simulink model "MicrostrainIMUTest02"  (R2013a)
settings: Solver=FixedStepDiscrete  StartTime=0.0  StopTime=inf  FixedStep=0.001  RelTol=1e-3
undefined symbols (not defined in the file or in its folder): IMU_Alignment_Params, KVHOrientationCal, m_XR17D15x, MicrostrainOrientationCal, standard, XOFF, XON
libraries: speedgoatlib x26, xpcethercatlib x25, xpcseriallib x13, simulink x5, dspswit3 x1, xpclib x1
(part 1 of 2)
settings Model: xpc_rtwmakecfg_data=_xpcethercatlib_  BufferReuse=off  Creator=bgbuss  LastModifiedBy=bgbuss
settings DataIOCC: LimitDataPoints=off
settings OptimizationCC: BlockReduction=off  OptimizeBlockIOStorage=off  BufferReuse=off  ExpressionFolding=off  LocalBlockOutputs=off
settings DebuggingCC: UnderspecifiedInitializationDetection=Simplified
settings HardwareCC: ProdIntDivRoundTo=Zero  ProdEndianess=LittleEndian  ProdHWDeviceType=Generic->32-bit x86 compatible
settings RTWCC: SystemTargetFile=xpctarget.tlc  TemplateMakefile=xpc_default_tmf  Description=xPC Target  ProcessScript=xpctarget_make_rtw_hook  RTWCompilerOptimization=On
settings xpcTargetCC: TargetFcnLib=ansi_tfl_table_tmw.mat  CodeReplacementLibrary=XPC_BLAS  ParMdlRefBuildCompliant=on  ConcurrentExecutionCompliant=on  CombineSignalStateStructs=off  MATLABClassNameForMDSCustomization=xpcAperiodicCustomization  GRTInterface=on  GenerateAllocFcn=off  RL32LogBufSizeModifier=100000000  xPCTaskExecutionProfile=off  xPCRL32EventNumber=5000  xPCisModelTimeout=off  xPCModelTimeoutSecs=20  xPCLoadParamSetFile=off  xPCConcurrentTasks=off  xPCEnableSFAnimation=off

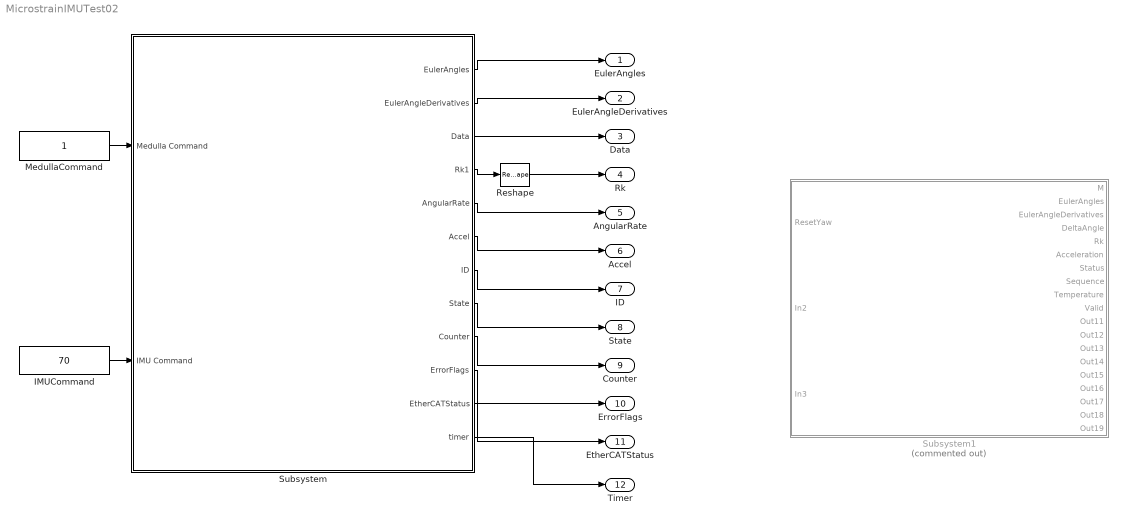
== system MicrostrainIMUTest02 ==
  IMUCommand : Constant  Value=70
  MedullaCommand : Constant
  Reshape : Reshape
  Subsystem : Subsystem
  Subsystem1 : Subsystem  Commented=on
  EulerAngles : Outport
  EulerAngleDerivatives : Outport  Port=2
  Data : Outport  Port=3
  Rk : Outport  Port=4
  AngularRate : Outport  Port=5
  Accel : Outport  Port=6
  ID : Outport  Port=7
  State : Outport  Port=8
  Counter : Outport  Port=9
  ErrorFlags : Outport  Port=10
  EtherCATStatus : Outport  Port=11
  Timer : Outport  Port=12
  wires:
  MedullaCommand/1 -> Subsystem/1(Medulla Command)
  IMUCommand/1 -> Subsystem/2(IMU Command)
  Subsystem/11(EtherCATStatus) -> EtherCATStatus/1
  Subsystem/1(EulerAngles) -> EulerAngles/1
  Subsystem/2(EulerAngleDerivatives) -> EulerAngleDerivatives/1
  Subsystem/3(Data) -> Data/1
  Subsystem/4(Rk1) -> Reshape/1
  Subsystem/5(AngularRate) -> AngularRate/1
  Subsystem/6(Accel) -> Accel/1
  Subsystem/7(ID) -> ID/1
  Subsystem/8(State) -> State/1
  Subsystem/9(Counter) -> Counter/1
  Subsystem/10(ErrorFlags) -> ErrorFlags/1
  Reshape/1 -> Rk/1
  Subsystem/12(timer) -> Timer/1

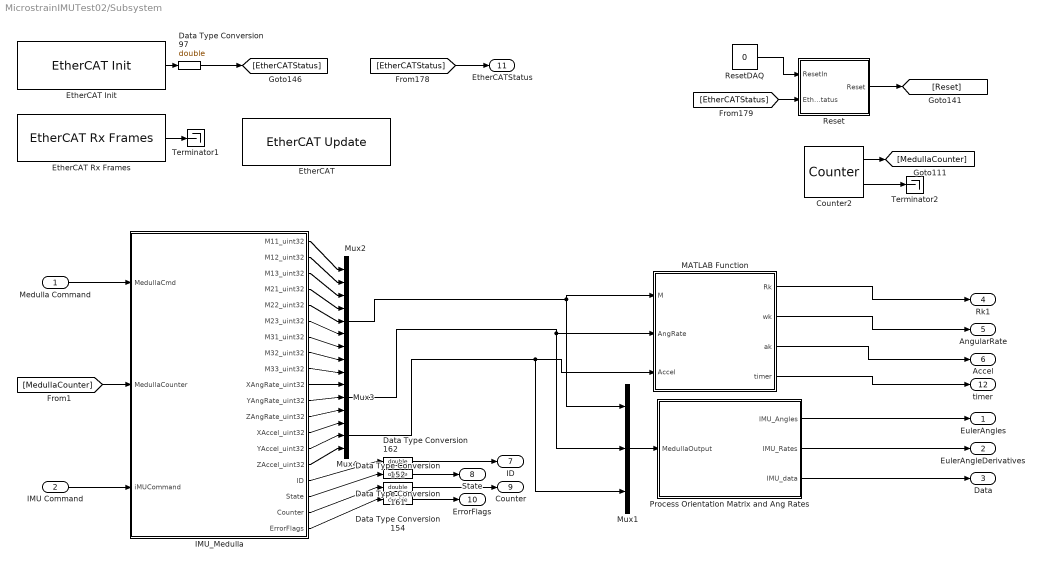
== system MicrostrainIMUTest02/Subsystem ==
  Medulla Command : Inport
  IMU Command : Inport  Port=2
  Counter2 : dspswit3/Counter  Direction=Up  CountEvent=Free running  CounterSize=User defined  MaxCount=65535  InitialCount=0  Output=Count and Hit  HitValue=32  ResetInput=off  SamplesPerFrame=1  Ts=.001  CntDtype=double  HitDtype=Logical
  Data Type Conversion{97,152,154,161..162} (5 alike) : DataTypeConversion  OutDataTypeStr=double
  EtherCAT : xpcethercatlib/EtherCAT Update   Priority=4  device_id=0  task_id_list=[1]  task_rates=[1]  task_priorities=[1500]
  EtherCAT Init : xpcethercatlib/EtherCAT Init   Priority=0  config_file='microstrain-imu-box07-eni.xml'  device_id=0  pci_bus=7  pci_slot=0  enaDC=on  errRptLevel=0  sample_time=0.001000
  EtherCAT Rx Frames : xpcethercatlib/EtherCAT Rx Frames   Priority=1  device_id=0  sample_time=0
  IMU_Medulla : Subsystem
  MATLAB Function : MATLAB Function  TreatAsAtomicUnit=on
  Mux1 : Mux  Inputs=3
  Mux2 : Mux  Inputs=9
  Mux3 : Mux  Inputs=3
  Mux4 : Mux  Inputs=3
  Process Orientation Matrix and Ang Rates : Subsystem
  Reset : Subsystem
  ResetDAQ : Constant  Value=0
  Terminator1 : Terminator
  Terminator2 : Terminator
  EulerAngles : Outport
  EulerAngleDerivatives : Outport  Port=2
  Data : Outport  Port=3
  Rk1 : Outport  Port=4
  AngularRate : Outport  Port=5
  Accel : Outport  Port=6
  ID : Outport  Port=7
  State : Outport  Port=8
  Counter : Outport  Port=9
  ErrorFlags : Outport  Port=10
  EtherCATStatus : Outport  Port=11
  timer : Outport  Port=12
  wires:
  IMU_Medulla/3(M13_uint32) -> Mux2/3
  IMU_Medulla/19(ErrorFlags) -> Data Type Conversion154/1
  IMU_Medulla/9(M33_uint32) -> Mux2/9
  IMU_Medulla/11(YAngRate_uint32) -> Mux3/2
  IMU_Medulla/15(ZAccel_uint32) -> Mux4/3
  [MedullaCounter] -> IMU_Medulla/2(MedullaCounter)
  IMU_Medulla/12(ZAngRate_uint32) -> Mux3/3
  IMU_Medulla/1(M11_uint32) -> Mux2/1
  IMU_Medulla/5(M22_uint32) -> Mux2/5
  IMU_Medulla/10(XAngRate_uint32) -> Mux3/1
  IMU_Medulla/14(YAccel_uint32) -> Mux4/2
  IMU_Medulla/13(XAccel_uint32) -> Mux4/1
  Data Type Conversion161/1 -> State/1
  IMU_Medulla/8(M32_uint32) -> Mux2/8
  Data Type Conversion162/1 -> ID/1
  IMU_Medulla/2(M12_uint32) -> Mux2/2
  IMU_Medulla/16(ID) -> Data Type Conversion162/1
  IMU_Medulla/6(M23_uint32) -> Mux2/6
  IMU_Medulla/4(M21_uint32) -> Mux2/4
  IMU_Medulla/7(M31_uint32) -> Mux2/7
  IMU_Medulla/18(Counter) -> Data Type Conversion152/1
  IMU_Medulla/17(State) -> Data Type Conversion161/1
  Mux3/1 -> Mux1/2, MATLAB Function/2(AngRate)
  Mux1/1 -> Process Orientation Matrix and Ang Rates/1(MedullaOutput)
  Process Orientation Matrix and Ang Rates/1(IMU_Angles) -> EulerAngles/1
  Process Orientation Matrix and Ang Rates/2(IMU_Rates) -> EulerAngleDerivatives/1
  Process Orientation Matrix and Ang Rates/3(IMU_data) -> Data/1
  [EtherCATStatus] -> EtherCATStatus/1
  ResetDAQ/1 -> Reset/1(ResetIn)
  Counter2/1 -> [MedullaCounter]
  [EtherCATStatus] -> Reset/2(EtherCATStatus)
  Reset/1(Reset) -> [Reset]
  Counter2/2 -> Terminator2/1
  Data Type Conversion97/1 -> [EtherCATStatus]
  EtherCAT Init/1 -> Data Type Conversion97/1
  EtherCAT Rx Frames/1 -> Terminator1/1
  Mux4/1 -> Mux1/3, MATLAB Function/3(Accel)
  Mux2/1 -> Mux1/1, MATLAB Function/1(M)
  Data Type Conversion152/1 -> Counter/1
  Data Type Conversion154/1 -> ErrorFlags/1
  Medulla Command/1 -> IMU_Medulla/1(MedullaCmd)
  IMU Command/1 -> IMU_Medulla/3(iMUCommand)
  MATLAB Function/1(Rk) -> Rk1/1
  MATLAB Function/2(wk) -> AngularRate/1
  MATLAB Function/3(ak) -> Accel/1
  MATLAB Function/4(timer) -> timer/1

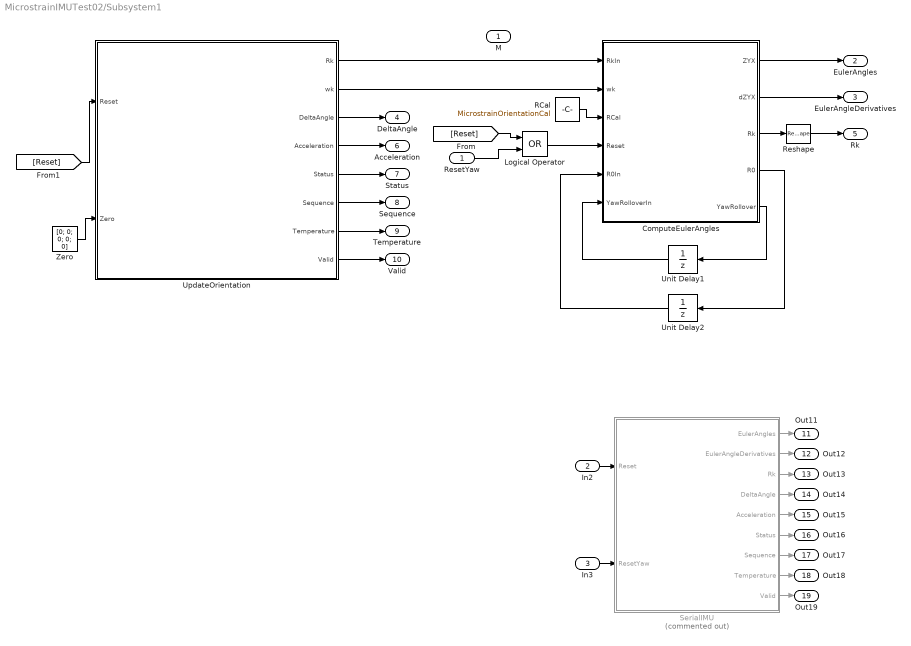
== system MicrostrainIMUTest02/Subsystem1 ==
  ResetYaw : Inport
  In2 : Inport  Port=2
  In3 : Inport  Port=3
  ComputeEulerAngles : MATLAB Function  TreatAsAtomicUnit=on
  Logical Operator : Logic  Operator=OR  AllPortsSameDT=off  OutDataTypeStr=boolean
  RCal : Constant  Value=MicrostrainOrientationCal
  Reshape : Reshape
  SerialIMU : Subsystem  Commented=on
  Unit Delay1 : UnitDelay  InitialCondition=[0; 0]  SampleTime=-1
  Unit Delay2 : UnitDelay  InitialCondition=zeros(3,3)  SampleTime=-1
  UpdateOrientation : Subsystem
  Zero : Constant  Value=[0; 0; 0; 0; 0]
  M : Outport
  EulerAngles : Outport  Port=2
  EulerAngleDerivatives : Outport  Port=3
  DeltaAngle : Outport  Port=4
  Rk : Outport  Port=5
  Acceleration : Outport  Port=6
  Status : Outport  Port=7
  Sequence : Outport  Port=8
  Temperature : Outport  Port=9
  Valid : Outport  Port=10
  Out11 : Outport  Port=11
  Out12 : Outport  Port=12
  Out13 : Outport  Port=13
  Out14 : Outport  Port=14
  Out15 : Outport  Port=15
  Out16 : Outport  Port=16
  Out17 : Outport  Port=17
  Out18 : Outport  Port=18
  Out19 : Outport  Port=19
  wires:
  SerialIMU/6(Status) -> Out16/1
  SerialIMU/8(Temperature) -> Out18/1
  In2/1 -> SerialIMU/1(Reset)
  SerialIMU/1(EulerAngles) -> Out11/1
  SerialIMU/3(Rk) -> Out13/1
  SerialIMU/5(Acceleration) -> Out15/1
  SerialIMU/2(EulerAngleDerivatives) -> Out12/1
  SerialIMU/7(Sequence) -> Out17/1
  In3/1 -> SerialIMU/2(ResetYaw)
  SerialIMU/9(Valid) -> Out19/1
  SerialIMU/4(DeltaAngle) -> Out14/1
  ComputeEulerAngles/1(ZYX) -> EulerAngles/1
  Logical Operator/1 -> ComputeEulerAngles/4(Reset)
  ResetYaw/1 -> Logical Operator/2
  Unit Delay1/1 -> ComputeEulerAngles/6(YawRolloverIn)
  ComputeEulerAngles/5(YawRollover) -> Unit Delay1/1
  UpdateOrientation/2(wk) -> ComputeEulerAngles/2(wk)
  UpdateOrientation/1(Rk) -> ComputeEulerAngles/1(RkIn)
  Reshape/1 -> Rk/1
  [Reset] -> Logical Operator/1
  ComputeEulerAngles/3(Rk) -> Reshape/1
  ComputeEulerAngles/4(R0) -> Unit Delay2/1
  Unit Delay2/1 -> ComputeEulerAngles/5(R0In)
  RCal/1 -> ComputeEulerAngles/3(RCal)
  [Reset] -> UpdateOrientation/1(Reset)
  Zero/1 -> UpdateOrientation/2(Zero)
  UpdateOrientation/3(DeltaAngle) -> DeltaAngle/1
  UpdateOrientation/6(Sequence) -> Sequence/1
  UpdateOrientation/5(Status) -> Status/1
  UpdateOrientation/4(Acceleration) -> Acceleration/1
  UpdateOrientation/7(Temperature) -> Temperature/1
  UpdateOrientation/8(Valid) -> Valid/1
  ComputeEulerAngles/2(dZYX) -> EulerAngleDerivatives/1

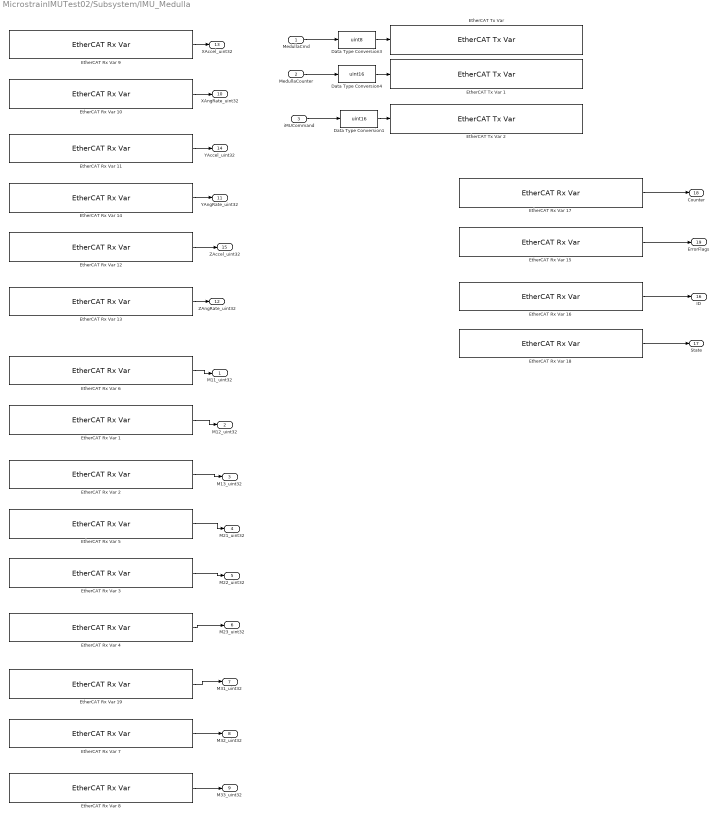
== system MicrostrainIMUTest02/Subsystem/IMU_Medulla ==
  MedullaCmd : Inport
  MedullaCounter : Inport  Port=2
  iMUCommand : Inport  Port=3
  Data Type Conversion1 : DataTypeConversion  OutDataTypeStr=uint16
  Data Type Conversion3 : DataTypeConversion  OutDataTypeStr=uint8
  Data Type Conversion4 : DataTypeConversion  OutDataTypeStr=uint16
  EtherCAT Rx Var 1 : xpcethercatlib/EtherCAT Rx Var   Priority=2  sig_name=Box 7 (ATRIAS 2.1 Microstrain IMU (Medulla 1.5)).M.M12  sig_offset=720  sig_type=uint32  type_size=32  sig_dim=1  device_id=0  sample_time=0.001000
  EtherCAT Rx Var 10 : xpcethercatlib/EtherCAT Rx Var   Priority=2  sig_name=Box 7 (ATRIAS 2.1 Microstrain IMU (Medulla 1.5)).Xaxes.XAngRate  sig_offset=496  sig_type=uint32  type_size=32  sig_dim=1  device_id=0  sample_time=0.001000
  EtherCAT Rx Var 11 : xpcethercatlib/EtherCAT Rx Var   Priority=2  sig_name=Box 7 (ATRIAS 2.1 Microstrain IMU (Medulla 1.5)).Yaxes.YAccel  sig_offset=592  sig_type=uint32  type_size=32  sig_dim=1  device_id=0  sample_time=0.001000
  EtherCAT Rx Var 12 : xpcethercatlib/EtherCAT Rx Var   Priority=2  sig_name=Box 7 (ATRIAS 2.1 Microstrain IMU (Medulla 1.5)).Zaxes.ZAccel  sig_offset=656  sig_type=uint32  type_size=32  sig_dim=1  device_id=0  sample_time=0.001000
  EtherCAT Rx Var 13 : xpcethercatlib/EtherCAT Rx Var   Priority=2  sig_name=Box 7 (ATRIAS 2.1 Microstrain IMU (Medulla 1.5)).Zaxes.ZAngRate  sig_offset=624  sig_type=uint32  type_size=32  sig_dim=1  device_id=0  sample_time=0.001000
  EtherCAT Rx Var 14 : xpcethercatlib/EtherCAT Rx Var   Priority=2  sig_name=Box 7 (ATRIAS 2.1 Microstrain IMU (Medulla 1.5)).Yaxes.YAngRate  sig_offset=560  sig_type=uint32  type_size=32  sig_dim=1  device_id=0  sample_time=0.001000
  EtherCAT Rx Var 15 : xpcethercatlib/EtherCAT Rx Var   Priority=2  sig_name=Box 7 (ATRIAS 2.1 Microstrain IMU (Medulla 1.5)).uController Status.Error Flags  sig_offset=488  sig_type=uint8  type_size=8  sig_dim=1  device_id=0  sample_time=0.001000
  EtherCAT Rx Var 16 : xpcethercatlib/EtherCAT Rx Var   Priority=2  sig_name=Box 7 (ATRIAS 2.1 Microstrain IMU (Medulla 1.5)).uController Status.ID  sig_offset=464  sig_type=uint8  type_size=8  sig_dim=1  device_id=0  sample_time=0.001000
  EtherCAT Rx Var 17 : xpcethercatlib/EtherCAT Rx Var   Priority=2  sig_name=Box 7 (ATRIAS 2.1 Microstrain IMU (Medulla 1.5)).uController Status.Counter  sig_offset=480  sig_type=uint8  type_size=8  sig_dim=1  device_id=0  sample_time=0.001000
  EtherCAT Rx Var 18 : xpcethercatlib/EtherCAT Rx Var   Priority=2  sig_name=Box 7 (ATRIAS 2.1 Microstrain IMU (Medulla 1.5)).uController Status.State  sig_offset=472  sig_type=uint8  type_size=8  sig_dim=1  device_id=0  sample_time=0.001000
  EtherCAT Rx Var 19 : xpcethercatlib/EtherCAT Rx Var   Priority=2  sig_name=Box 7 (ATRIAS 2.1 Microstrain IMU (Medulla 1.5)).M.M31  sig_offset=880  sig_type=uint32  type_size=32  sig_dim=1  device_id=0  sample_time=0.001000
  EtherCAT Rx Var 2 : xpcethercatlib/EtherCAT Rx Var   Priority=2  sig_name=Box 7 (ATRIAS 2.1 Microstrain IMU (Medulla 1.5)).M.M13  sig_offset=752  sig_type=uint32  type_size=32  sig_dim=1  device_id=0  sample_time=0.001000
  EtherCAT Rx Var 3 : xpcethercatlib/EtherCAT Rx Var   Priority=2  sig_name=Box 7 (ATRIAS 2.1 Microstrain IMU (Medulla 1.5)).M.M22  sig_offset=816  sig_type=uint32  type_size=32  sig_dim=1  device_id=0  sample_time=0.001000
  EtherCAT Rx Var 4 : xpcethercatlib/EtherCAT Rx Var   Priority=2  sig_name=Box 7 (ATRIAS 2.1 Microstrain IMU (Medulla 1.5)).M.M23  sig_offset=848  sig_type=uint32  type_size=32  sig_dim=1  device_id=0  sample_time=0.001000
  EtherCAT Rx Var 5 : xpcethercatlib/EtherCAT Rx Var   Priority=2  sig_name=Box 7 (ATRIAS 2.1 Microstrain IMU (Medulla 1.5)).M.M21  sig_offset=784  sig_type=uint32  type_size=32  sig_dim=1  device_id=0  sample_time=0.001000
  EtherCAT Rx Var 6 : xpcethercatlib/EtherCAT Rx Var   Priority=2  sig_name=Box 7 (ATRIAS 2.1 Microstrain IMU (Medulla 1.5)).M.M11  sig_offset=688  sig_type=uint32  type_size=32  sig_dim=1  device_id=0  sample_time=0.001000
  EtherCAT Rx Var 7 : xpcethercatlib/EtherCAT Rx Var   Priority=2  sig_name=Box 7 (ATRIAS 2.1 Microstrain IMU (Medulla 1.5)).M.M32  sig_offset=912  sig_type=uint32  type_size=32  sig_dim=1  device_id=0  sample_time=0.001000
  EtherCAT Rx Var 8 : xpcethercatlib/EtherCAT Rx Var   Priority=2  sig_name=Box 7 (ATRIAS 2.1 Microstrain IMU (Medulla 1.5)).M.M33  sig_offset=944  sig_type=uint32  type_size=32  sig_dim=1  device_id=0  sample_time=0.001000
  EtherCAT Rx Var 9 : xpcethercatlib/EtherCAT Rx Var   Priority=2  sig_name=Box 7 (ATRIAS 2.1 Microstrain IMU (Medulla 1.5)).Xaxes.XAccel  sig_offset=528  sig_type=uint32  type_size=32  sig_dim=1  device_id=0  sample_time=0.001000
  "EtherCAT Tx Var " : xpcethercatlib/EtherCAT Tx Var   Priority=3  sig_name=Box 7 (ATRIAS 2.1 Microstrain IMU (Medulla 1.5)).uControllerInput.Command  sig_offset=464  sig_type=uint8  type_size=8  sig_dim=1  device_id=0  sample_time=0.001000
  EtherCAT Tx Var 1 : xpcethercatlib/EtherCAT Tx Var   Priority=3  sig_name=Box 7 (ATRIAS 2.1 Microstrain IMU (Medulla 1.5)).uControllerInput.Counter  sig_offset=472  sig_type=uint16  type_size=16  sig_dim=1  device_id=0  sample_time=0.001000
  EtherCAT Tx Var 2 : xpcethercatlib/EtherCAT Tx Var   Priority=3  sig_name=Box 7 (ATRIAS 2.1 Microstrain IMU (Medulla 1.5)).uControllerInput.IMU_cmd  sig_offset=488  sig_type=uint16  type_size=16  sig_dim=1  device_id=0  sample_time=0.001000
  M11_uint32 : Outport
  M12_uint32 : Outport  Port=2
  M13_uint32 : Outport  Port=3
  M21_uint32 : Outport  Port=4
  M22_uint32 : Outport  Port=5
  M23_uint32 : Outport  Port=6
  M31_uint32 : Outport  Port=7
  M32_uint32 : Outport  Port=8
  M33_uint32 : Outport  Port=9
  XAngRate_uint32 : Outport  Port=10
  YAngRate_uint32 : Outport  Port=11
  ZAngRate_uint32 : Outport  Port=12
  XAccel_uint32 : Outport  Port=13
  YAccel_uint32 : Outport  Port=14
  ZAccel_uint32 : Outport  Port=15
  ID : Outport  Port=16
  State : Outport  Port=17
  Counter : Outport  Port=18
  ErrorFlags : Outport  Port=19
  wires:
  EtherCAT Rx Var 9/1 -> XAccel_uint32/1
  EtherCAT Rx Var 10/1 -> XAngRate_uint32/1
  EtherCAT Rx Var 11/1 -> YAccel_uint32/1
  EtherCAT Rx Var 14/1 -> YAngRate_uint32/1
  EtherCAT Rx Var 12/1 -> ZAccel_uint32/1
  EtherCAT Rx Var 13/1 -> ZAngRate_uint32/1
  EtherCAT Rx Var 6/1 -> M11_uint32/1
  EtherCAT Rx Var 1/1 -> M12_uint32/1
  EtherCAT Rx Var 2/1 -> M13_uint32/1
  EtherCAT Rx Var 5/1 -> M21_uint32/1
  EtherCAT Rx Var 3/1 -> M22_uint32/1
  EtherCAT Rx Var 4/1 -> M23_uint32/1
  EtherCAT Rx Var 19/1 -> M31_uint32/1
  EtherCAT Rx Var 7/1 -> M32_uint32/1
  EtherCAT Rx Var 8/1 -> M33_uint32/1
  Data Type Conversion3/1 -> "EtherCAT Tx Var "/1
  Data Type Conversion4/1 -> EtherCAT Tx Var 1/1
  MedullaCmd/1 -> Data Type Conversion3/1
  MedullaCounter/1 -> Data Type Conversion4/1
  iMUCommand/1 -> Data Type Conversion1/1
  Data Type Conversion1/1 -> EtherCAT Tx Var 2/1
  EtherCAT Rx Var 17/1 -> Counter/1
  EtherCAT Rx Var 15/1 -> ErrorFlags/1
  EtherCAT Rx Var 16/1 -> ID/1
  EtherCAT Rx Var 18/1 -> State/1

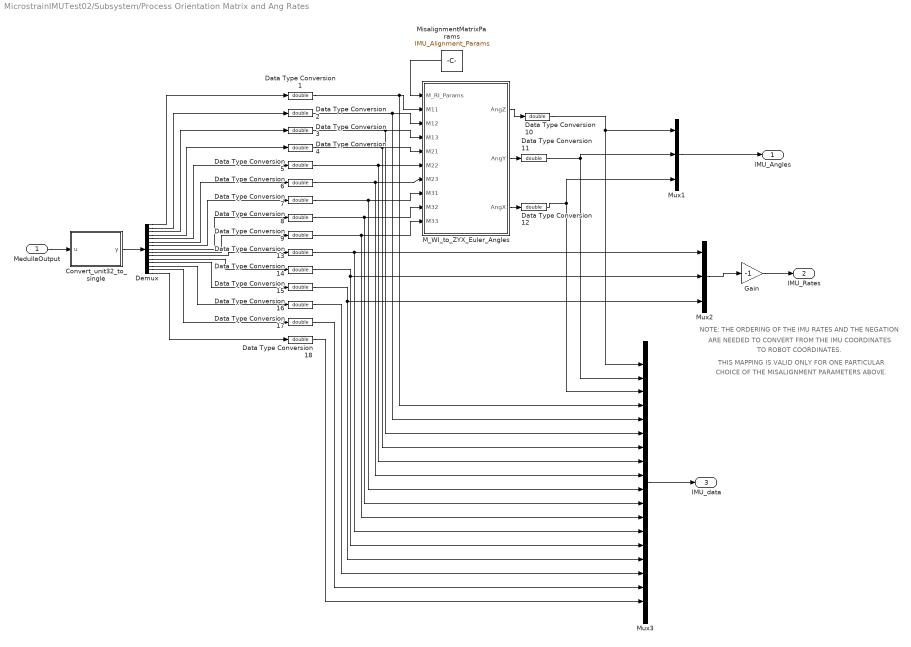
== system MicrostrainIMUTest02/Subsystem/Process Orientation Matrix and Ang Rates ==
  note: NOTE: THE ORDERING OF THE IMU RATES AND THE NEGATION
  note: ARE NEEDED TO CONVERT FROM THE IMU COORDINATES
  note: TO ROBOT COORDINATES.
  note: THIS MAPPING IS VALID ONLY FOR ONE PARTICULAR
  note: CHOICE OF THE MISALIGNMENT PARAMETERS ABOVE.
  MedullaOutput : Inport
  Convert_unit32_to_single : MATLAB Function  TreatAsAtomicUnit=on
  Data Type Conversion{1..18} (18 alike) : DataTypeConversion  OutDataTypeStr=double
  Demux : Demux  Outputs=15
  Gain : Gain  Gain=-1
  M_WI_to_ZYX_Euler_Angles : MATLAB Function  TreatAsAtomicUnit=on
  MisalignmentMatrixParams : Constant  Value=IMU_Alignment_Params
  Mux1 : Mux  Inputs=3
  Mux2 : Mux  Inputs=3
  Mux3 : Mux  Inputs=18
  IMU_Angles : Outport
  IMU_Rates : Outport  Port=2
  IMU_data : Outport  Port=3
  wires:
  Mux3/1 -> IMU_data/1
  Mux1/1 -> IMU_Angles/1
  Data Type Conversion16/1 -> Mux3/16
  Data Type Conversion17/1 -> Mux3/17
  Data Type Conversion18/1 -> Mux3/18
  Demux/15 -> Data Type Conversion18/1
  Demux/14 -> Data Type Conversion17/1
  Demux/13 -> Data Type Conversion16/1
  Demux/12 -> Data Type Conversion15/1
  Demux/11 -> Data Type Conversion14/1
  Demux/10 -> Data Type Conversion13/1
  Demux/9 -> Data Type Conversion9/1
  Demux/8 -> Data Type Conversion8/1
  Demux/7 -> Data Type Conversion7/1
  Demux/6 -> Data Type Conversion6/1
  Demux/5 -> Data Type Conversion5/1
  Demux/4 -> Data Type Conversion4/1
  Demux/3 -> Data Type Conversion3/1
  Demux/2 -> Data Type Conversion2/1
  Demux/1 -> Data Type Conversion1/1
  MisalignmentMatrixParams/1 -> M_WI_to_ZYX_Euler_Angles/1(M_RI_Params)
  Data Type Conversion15/1 -> Mux3/15, Mux2/3
  Data Type Conversion14/1 -> Mux3/14, Mux2/2
  Data Type Conversion13/1 -> Mux3/13, Mux2/1
  Data Type Conversion12/1 -> Mux3/3, Mux1/3
  Data Type Conversion11/1 -> Mux3/2, Mux1/2
  Data Type Conversion10/1 -> Mux3/1, Mux1/1
  Data Type Conversion9/1 -> Mux3/12, M_WI_to_ZYX_Euler_Angles/10(M33)
  Data Type Conversion8/1 -> Mux3/11, M_WI_to_ZYX_Euler_Angles/9(M32)
  Data Type Conversion7/1 -> Mux3/10, M_WI_to_ZYX_Euler_Angles/8(M31)
  Data Type Conversion6/1 -> Mux3/9, M_WI_to_ZYX_Euler_Angles/7(M23)
  Data Type Conversion5/1 -> Mux3/8, M_WI_to_ZYX_Euler_Angles/6(M22)
  Data Type Conversion4/1 -> Mux3/7, M_WI_to_ZYX_Euler_Angles/5(M21)
  Data Type Conversion3/1 -> Mux3/6, M_WI_to_ZYX_Euler_Angles/4(M13)
  Data Type Conversion2/1 -> Mux3/5, M_WI_to_ZYX_Euler_Angles/3(M12)
  Data Type Conversion1/1 -> Mux3/4, M_WI_to_ZYX_Euler_Angles/2(M11)
  M_WI_to_ZYX_Euler_Angles/3(AngX) -> Data Type Conversion12/1
  M_WI_to_ZYX_Euler_Angles/2(AngY) -> Data Type Conversion11/1
  M_WI_to_ZYX_Euler_Angles/1(AngZ) -> Data Type Conversion10/1
  MedullaOutput/1 -> Convert_unit32_to_single/1(u)
  Convert_unit32_to_single/1(y) -> Demux/1
  Mux2/1 -> Gain/1
  Gain/1 -> IMU_Rates/1

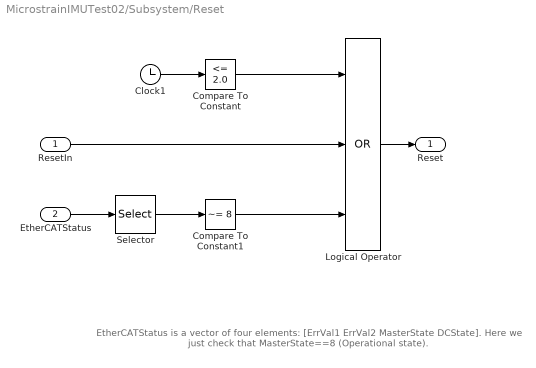
== system MicrostrainIMUTest02/Subsystem/Reset ==
  note: EtherCATStatus is a vector of four elements:
      | [ErrVal1 ErrVal2 MasterState DCState].
      | Here we just check that MasterState==8 (Operational state).
  ResetIn : Inport
  EtherCATStatus : Inport  Port=2
  Clock1 : Clock
  Compare To Constant : simulink/Logic and Bit Operations/Compare To Constant  relop=<=  const=2.0  OutDataTypeStr=uint8
  Compare To Constant1 : simulink/Logic and Bit Operations/Compare To Constant  relop=~=  const=8  OutDataTypeStr=uint8
  Logical Operator : Logic  Operator=OR  Inputs=3  AllPortsSameDT=off  OutDataTypeStr=boolean
  Selector : Selector  InputPortWidth=4  IndexOptions=Index vector (dialog)  Indices=[3]  OutputSizes=1
  Reset : Outport
  wires:
  Selector/1 -> Compare To Constant1/1
  EtherCATStatus/1 -> Selector/1
  Compare To Constant1/1 -> Logical Operator/3
  Clock1/1 -> Compare To Constant/1
  Compare To Constant/1 -> Logical Operator/1
  ResetIn/1 -> Logical Operator/2
  Logical Operator/1 -> Reset/1

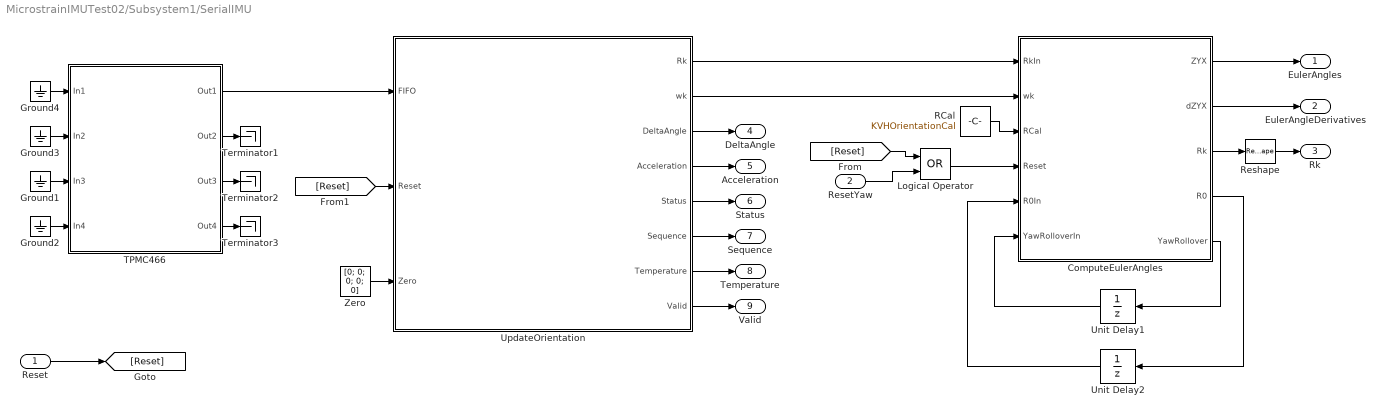
== system MicrostrainIMUTest02/Subsystem1/SerialIMU ==
  Reset : Inport
  ResetYaw : Inport  Port=2
  ComputeEulerAngles : MATLAB Function  TreatAsAtomicUnit=on
  Ground{1..4} (4 alike) : Ground
  Logical Operator : Logic  Operator=OR  AllPortsSameDT=off  OutDataTypeStr=boolean
  RCal : Constant  Value=KVHOrientationCal
  Reshape : Reshape
  TPMC466 : Subsystem  InitFcn=m_XR17D15x(3);  mask(RS232 Send Receive){group=Board Setup, port=1, irqnum=9, slot=[4 5], transceiver1=RS422, standard1=on, baud1=921600, bauddivisor1=1, sampling1=16x (standard), prescale1=off, parity1=None, ndata1=8, nstop1=1, rlevel1=quarter full (16), hwmode1=none, swmode1=none, xonchar1=17, xoffchar1=19, rs485auto1=off, rs485delay1=1, xmtfifosize1=1024, xmtdatatype1=8 bit uint null terminated, rcvfifosize1=1024, transceiver2=RS485 half-duplex, standard2=on, baud2=2764800, bauddivisor2=1, sampling2=16x (standard), prescale2=off, parity2=None, ndata2=8, nstop2=1, rlevel2=quarter full (16), hwmode2=none, swmode2=XON/XOFF, xonchar2=17, xoffchar2=19, rs485auto2=on, rs485delay2=1, xmtfifosize2=1024, xmtdatatype2=8 bit uint null terminated, rcvfifosize2=1024, transceiver3=RS485 half-duplex, standard3=on, baud3=115200, bauddivisor3=1, sampling3=16x (standard), prescale3=off, parity3=None, ndata3=8, nstop3=1, rlevel3=half full (32), hwmode3=none, swmode3=none, xonchar3=17, xoffchar3=19, rs485auto3=off, rs485delay3=0, xmtfifosize3=1024, xmtdatatype3=8 bit uint null terminated, rcvfifosize3=1024, transceiver4=RS485 half-duplex, standard4=on, baud4=115200, bauddivisor4=1, sampling4=16x (standard), prescale4=off, parity4=None, ndata4=8, nstop4=1, rlevel4=half full (32), hwmode4=none, swmode4=none, xonchar4=17, xoffchar4=19, rs485auto4=off, rs485delay4=0, xmtfifosize4=1024, xmtdatatype4=8 bit uint null terminated, rcvfifosize4=1024}
      mask prompts: group "Parameter group:"; port "Port to modify:"; irqnum "IRQ number:"; slot "PCI slot (-1: autosearch):"; transceiver1 "Transceiver setup:"; standard1 "Use standard baud rates (16x, no prescaling)"; baud1 "Standard baud rate:"; bauddivisor1 "Baud rate divisor (non-standard baud rates):"; sampling1 "Sampling rate (non-standard baud rates):"; prescale1 "Prescale by 4 (non-standard baud rates)"; parity1 "Parity:"; ndata1 "Data bits:"; nstop1 "Stop bits:"; rlevel1 "Receive FIFO interrupt level:"; hwmode1 "Hardware handshake:"; swmode1 "Software handshake:"; xonchar1 "XON character:"; xoffchar1 "XOFF character:"; rs485auto1 "RS485 auto turnaround:"; rs485delay1 "RS485 turnaround delay [0,15]"; xmtfifosize1 "Transmit software FIFO size:"; xmtdatatype1 "Transmit FIFO data type:"; rcvfifosize1 "Receive software FIFO size:"; transceiver2 "Transceiver setup:"; standard2 "Use standard baud rates (16x, no prescaling)"; baud2 "Standard baud rate:"; bauddivisor2 "Baud rate divisor (non-standard baud rates):"; sampling2 "Sampling rate (non-standard baud rates):"; prescale2 "Prescale by 4 (non-standard baud rates)"; parity2 "Parity:"; ndata2 "Data bits:"; nstop2 "Stop bits:"; rlevel2 "Receive FIFO interrupt level:"; hwmode2 "Hardware handshake:"; swmode2 "Software handshake:"; xonchar2 "XON character:"; xoffchar2 "XOFF character:"; rs485auto2 "RS485 auto turnaround:"; rs485delay2 "RS485 turnaround delay [0,15]"; xmtfifosize2 "Transmit software FIFO size:"; xmtdatatype2 "Transmit FIFO data type:"; rcvfifosize2 "Receive software FIFO size:"; transceiver3 "Transceiver setup:"; standard3 "Use standard baud rates (16x, no prescaling)"; baud3 "Standard baud rate:"; bauddivisor3 "Baud rate divisor (non-standard baud rates):"; sampling3 "Sampling rate (non-standard baud rates):"; prescale3 "Prescale by 4 (non-standard baud rates)"; parity3 "Parity:"; ndata3 "Data bits:"; nstop3 "Stop bits:"; rlevel3 "Receive FIFO interrupt level:"; hwmode3 "Hardware handshake:"; swmode3 "Software handshake:"; xonchar3 "XON character:"; xoffchar3 "XOFF character:"; rs485auto3 "RS485 auto turnaround:"; rs485delay3 "RS485 turnaround delay [0,15]"; xmtfifosize3 "Transmit software FIFO size:"; xmtdatatype3 "Transmit FIFO data type:"; rcvfifosize3 "Receive software FIFO size:"; transceiver4 "Transceiver setup:"; standard4 "Use standard baud rates (16x, no prescaling)"; baud4 "Standard baud rate:"; bauddivisor4 "Baud rate divisor (non-standard baud rates):"; sampling4 "Sampling rate (non-standard baud rates):"; prescale4 "Prescale by 4 (non-standard baud rates)"; parity4 "Parity:"; ndata4 "Data bits:"; nstop4 "Stop bits:"; rlevel4 "Receive FIFO interrupt level:"; hwmode4 "Hardware handshake:"; swmode4 "Software handshake:"; xonchar4 "XON character:"; xoffchar4 "XOFF character:"; rs485auto4 "RS485 auto turnaround:"; rs485delay4 "RS485 turnaround delay [0,15]"; xmtfifosize4 "Transmit software FIFO size:"; xmtdatatype4 "Transmit FIFO data type:"; rcvfifosize4 "Receive software FIFO size:"
      mask help:
      | PMC521
      | Acromag
      | EIA/TIA-422B Send Receive Subsystem
      mask init:
      | brdslot = slot;
      | m_tews_XR17D15x(1, 4);
      mask Help: helpview(fullfile(docroot, 'mapfiles', 'xpc.map'), 'Commtech_Subsystem')
      mask TypeOptions group: Board Setup | Basic Setup | FIFO Setup
      mask Callback group: m_tews_XR17D15x(2, 4);
      mask TypeOptions port: 1 | 2 | 3 | 4
      mask Callback port: m_tews_XR17D15x(2, 4);
      mask TypeOptions transceiver1: RS232 (max 921.6kb/s) | RS422 | RS422 multidrop | RS485 full-duplex | RS485 half-duplex
      mask TypeOptions baud1: 2764800 | 1382400 | 921600 | 460800 | 230400 | 115200 | 57600 | 38400 | 19200 | 9600 | 4800 | 2400 | 1200 | 600 | 400
      mask TypeOptions sampling1: 8x | 16x (standard)
      mask TypeOptions parity1: None | Even | Odd | Mark | Space
      mask TypeOptions ndata1: 5 | 6 | 7 | 8
      mask TypeOptions nstop1: 1 | 2
      mask TypeOptions rlevel1: 1 | quarter full (16) | half full (32) | almost full (56)
      mask TypeOptions hwmode1: RTS/CTS | none
      mask TypeOptions swmode1: XON/XOFF | none
      mask TypeOptions xmtdatatype1: count+32 bit int | count+32 bit uint | count+16 bit int | count+16 bit uint | 8 bit int null terminated | 8 bit uint null terminated
      mask TypeOptions transceiver2: RS232 (max 921.6kb/s) | RS422 | RS422 multidrop | RS485 full-duplex | RS485 half-duplex
      mask TypeOptions baud2: 2764800 | 1382400 | 921600 | 460800 | 230400 | 115200 | 57600 | 38400 | 19200 | 9600 | 4800 | 2400 | 1200 | 600 | 400
      mask TypeOptions sampling2: 8x | 16x (standard)
      mask TypeOptions parity2: None | Even | Odd | Mark | Space
      mask TypeOptions ndata2: 5 | 6 | 7 | 8
      mask TypeOptions nstop2: 1 | 2
      mask TypeOptions rlevel2: 1 | quarter full (16) | half full (32) | almost full (56)
      mask TypeOptions hwmode2: RTS/CTS | none
      mask TypeOptions swmode2: XON/XOFF | none
      mask TypeOptions xmtdatatype2: count+32 bit int | count+32 bit uint | count+16 bit int | count+16 bit uint | 8 bit int null terminated | 8 bit uint null terminated
      mask TypeOptions transceiver3: RS232 (max 921.6kb/s) | RS422 | RS422 multidrop | RS485 full-duplex | RS485 half-duplex
      mask TypeOptions baud3: 2764800 | 1382400 | 921600 | 460800 | 230400 | 115200 | 57600 | 38400 | 19200 | 9600 | 4800 | 2400 | 1200 | 600 | 400
      mask TypeOptions sampling3: 8x | 16x (standard)
      mask TypeOptions parity3: None | Even | Odd | Mark | Space
      mask TypeOptions ndata3: 5 | 6 | 7 | 8
      mask TypeOptions nstop3: 1 | 2
      mask TypeOptions rlevel3: 1 | quarter full (16) | half full (32) | almost full (56)
      mask TypeOptions hwmode3: RTS/CTS | none
      mask TypeOptions swmode3: XON/XOFF | none
      mask TypeOptions xmtdatatype3: count+32 bit int | count+32 bit uint | count+16 bit int | count+16 bit uint | 8 bit int null terminated | 8 bit uint null terminated
      mask TypeOptions transceiver4: RS232 (max 921.6kb/s) | RS422 | RS422 multidrop | RS485 full-duplex | RS485 half-duplex
      mask TypeOptions baud4: 2764800 | 1382400 | 921600 | 460800 | 230400 | 115200 | 57600 | 38400 | 19200 | 9600 | 4800 | 2400 | 1200 | 600 | 400
      mask TypeOptions sampling4: 8x | 16x (standard)
      mask TypeOptions parity4: None | Even | Odd | Mark | Space
      mask TypeOptions ndata4: 5 | 6 | 7 | 8
      mask TypeOptions nstop4: 1 | 2
      mask TypeOptions rlevel4: 1 | quarter full (16) | half full (32) | almost full (56)
      mask TypeOptions hwmode4: RTS/CTS | none
      mask TypeOptions swmode4: XON/XOFF | none
      mask TypeOptions xmtdatatype4: count+32 bit int | count+32 bit uint | count+16 bit int | count+16 bit uint | 8 bit int null terminated | 8 bit uint null terminated
      mask Display:
      | disp('TEWS\nTPMC466\nRS232/422/485\nSend\nReceive');
      | port_label( 'input', 1, 'XMT1' );
      | port_label( 'input', 2, 'XMT2' );
      | port_label( 'input', 3, 'XMT3' );
      | port_label( 'input', 4, 'XMT4' );
      | 
      | port_label( 'output', 1, 'FIFO1' );
      | port_label( 'output', 2, 'FIFO2' );
      | port_label( 'output', 3, 'FIFO3' );
      | port_label( 'output', 4, 'FIFO4' );
  Terminator1 : Terminator
  Terminator2 : Terminator
  Terminator3 : Terminator
  Unit Delay1 : UnitDelay  InitialCondition=[0; 0]  SampleTime=-1
  Unit Delay2 : UnitDelay  InitialCondition=zeros(3,3)  SampleTime=-1
  UpdateOrientation : Subsystem
  Zero : Constant  Value=[0; 0; 0; 0; 0]
  EulerAngles : Outport
  EulerAngleDerivatives : Outport  Port=2
  Rk : Outport  Port=3
  DeltaAngle : Outport  Port=4
  Acceleration : Outport  Port=5
  Status : Outport  Port=6
  Sequence : Outport  Port=7
  Temperature : Outport  Port=8
  Valid : Outport  Port=9
  wires:
  RCal/1 -> ComputeEulerAngles/3(RCal)
  Unit Delay2/1 -> ComputeEulerAngles/5(R0In)
  ComputeEulerAngles/1(ZYX) -> EulerAngles/1
  ComputeEulerAngles/4(R0) -> Unit Delay2/1
  ComputeEulerAngles/3(Rk) -> Reshape/1
  [Reset] -> Logical Operator/1
  Reshape/1 -> Rk/1
  Ground4/1 -> TPMC466/1(In1)
  Ground3/1 -> TPMC466/2(In2)
  Ground1/1 -> TPMC466/3(In3)
  Ground2/1 -> TPMC466/4(In4)
  TPMC466/3(Out3) -> Terminator2/1
  TPMC466/4(Out4) -> Terminator3/1
  TPMC466/2(Out2) -> Terminator1/1
  TPMC466/1(Out1) -> UpdateOrientation/1(FIFO)
  Reset/1 -> [Reset]
  [Reset] -> UpdateOrientation/2(Reset)
  Zero/1 -> UpdateOrientation/3(Zero)
  UpdateOrientation/1(Rk) -> ComputeEulerAngles/1(RkIn)
  UpdateOrientation/3(DeltaAngle) -> DeltaAngle/1
  UpdateOrientation/6(Sequence) -> Sequence/1
  UpdateOrientation/5(Status) -> Status/1
  UpdateOrientation/4(Acceleration) -> Acceleration/1
  UpdateOrientation/7(Temperature) -> Temperature/1
  UpdateOrientation/8(Valid) -> Valid/1
  UpdateOrientation/2(wk) -> ComputeEulerAngles/2(wk)
  ComputeEulerAngles/2(dZYX) -> EulerAngleDerivatives/1
  ComputeEulerAngles/5(YawRollover) -> Unit Delay1/1
  Unit Delay1/1 -> ComputeEulerAngles/6(YawRolloverIn)
  ResetYaw/1 -> Logical Operator/2
  Logical Operator/1 -> ComputeEulerAngles/4(Reset)

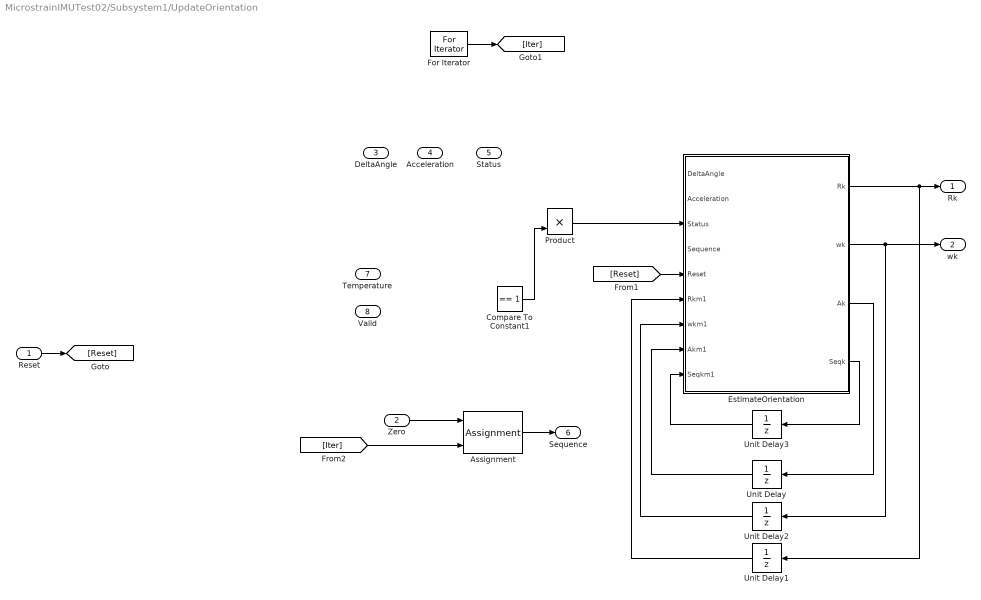
== system MicrostrainIMUTest02/Subsystem1/UpdateOrientation ==
  Reset : Inport
  Zero : Inport  Port=2
  Assignment : Assignment  IndexOptions=Index vector (port)  Indices=1  OutputSizes=1
  Compare To Constant1 : simulink/Logic and Bit Operations/Compare To Constant  relop===  const=1  OutDataTypeStr=uint8
  EstimateOrientation : MATLAB Function  TreatAsAtomicUnit=on
  For Iterator : ForIterator
  Product : Product  RndMeth=Zero
  Unit Delay : UnitDelay  InitialCondition=[0; 0; 0]  SampleTime=-1
  Unit Delay1 : UnitDelay  InitialCondition=zeros(3,3)  SampleTime=-1
  Unit Delay2 : UnitDelay  InitialCondition=[0; 0; 0]  SampleTime=-1
  Unit Delay3 : UnitDelay  SampleTime=-1
  Rk : Outport  InitialOutput=zeros(3,3)
  wk : Outport  Port=2  InitialOutput=zeros(3,1)
  DeltaAngle : Outport  Port=3  InitialOutput=zeros(3,1)
  Acceleration : Outport  Port=4  InitialOutput=zeros(3,1)
  Status : Outport  Port=5  InitialOutput=0
  Sequence : Outport  Port=6  InitialOutput=[0; 0; 0; 0; 0]
  Temperature : Outport  Port=7  InitialOutput=0
  Valid : Outport  Port=8  InitialOutput=0
  wires:
  ? -> Acceleration/1, EstimateOrientation/2(Acceleration)
  ? -> DeltaAngle/1, EstimateOrientation/1(DeltaAngle)
  ? -> Status/1, Product/1
  ? -> Assignment/2, EstimateOrientation/4(Sequence)
  ? -> Temperature/1
  ? -> Valid/1, Compare To Constant1/1
  EstimateOrientation/3(Ak) -> Unit Delay/1
  Unit Delay/1 -> EstimateOrientation/8(Akm1)
  EstimateOrientation/1(Rk) -> Rk/1, Unit Delay1/1
  Unit Delay1/1 -> EstimateOrientation/6(Rkm1)
  [Reset] -> EstimateOrientation/5(Reset)
  Product/1 -> EstimateOrientation/3(Status)
  Compare To Constant1/1 -> Product/2
  EstimateOrientation/4(Seqk) -> Unit Delay3/1
  Unit Delay3/1 -> EstimateOrientation/9(Seqkm1)
  Reset/1 -> [Reset]
  [Iter] -> Assignment/3
  Assignment/1 -> Sequence/1
  Zero/1 -> Assignment/1
  For Iterator/1 -> [Iter]
  EstimateOrientation/2(wk) -> wk/1, Unit Delay2/1
  Unit Delay2/1 -> EstimateOrientation/7(wkm1)

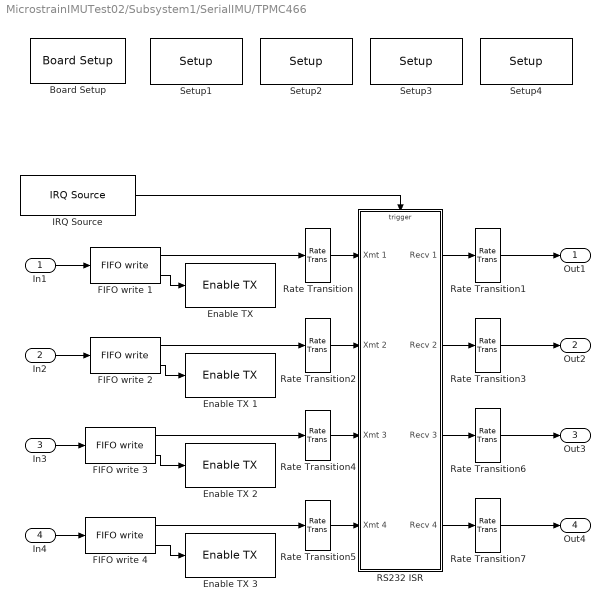
== system MicrostrainIMUTest02/Subsystem1/SerialIMU/TPMC466 ==
  In1 : Inport
  In2 : Inport  Port=2
  In3 : Inport  Port=3
  In4 : Inport  Port=4
  Board Setup : speedgoatlib/IO503/TEWS TPMC466 Internal blocks/Board Setup  irqnum=9  slot=brdslot
  "Enable TX " : speedgoatlib/IO503/TEWS TPMC466 Internal blocks/Enable TX   port=1  slot=brdslot
  Enable TX 1 : speedgoatlib/IO503/TEWS TPMC466 Internal blocks/Enable TX   port=2  slot=brdslot
  Enable TX 2 : speedgoatlib/IO503/TEWS TPMC466 Internal blocks/Enable TX   port=3  slot=brdslot
  Enable TX 3 : speedgoatlib/IO503/TEWS TPMC466 Internal blocks/Enable TX   port=4  slot=brdslot
  FIFO write 1 : xpcseriallib/FIFO write   size=1024  inputtype=8 bit uint null terminated  present=on  sampletime=-1  id=XMT channel 1, IRQ 9
  FIFO write 2 : xpcseriallib/FIFO write   size=1024  inputtype=8 bit uint null terminated  present=on  sampletime=-1  id=XMT channel 2, IRQ 9
  FIFO write 3 : xpcseriallib/FIFO write   size=1024  inputtype=8 bit uint null terminated  present=on  sampletime=-1  id=XMT channel 3, IRQ 9
  FIFO write 4 : xpcseriallib/FIFO write   size=1024  inputtype=8 bit uint null terminated  present=on  sampletime=-1  id=XMT channel 4, IRQ 9
  IRQ Source : xpclib/Asynchronous Event/IRQ Source  irqNo=9  preempt=off  b_type=None/Other  slot=brdslot
  RS232 ISR : Subsystem  TreatAsAtomicUnit=on  mask(RS232 ISR){slot=brdslot}
      mask help:
      | PMC521
      | Acromag
      | Interrupt Service Routine
      mask init:
      | subslot = slot;
      mask Display:
      | disp('PMC521\nAcromag\nISR');
      | port_label('input', 1, 'XMT1');
      | port_label('input', 2, 'XMT2');
      | port_label('input', 3, 'XMT3');
      | port_label('input', 4, 'XMT4');
      | port_label('input', 5, 'XMT5');
      | port_label('input', 6, 'XMT6');
      | port_label('input', 7, 'XMT7');
      | port_label('input', 8, 'XMT8');
      | port_label('output', 1, 'RCV1');
      | port_label('output', 2, 'RCV2');
      | port_label('output', 3, 'RCV3');
      | port_label('output', 4, 'RCV4');
      | port_label('output', 5, 'RCV5');
      | port_label('output', 6, 'RCV6');
      | port_label('output', 7, 'RCV7');
      | port_label('output', 8, 'RCV8');
  Rate Transition{,2,4..5} (4 alike) : RateTransition  Integrity=off  Deterministic=off
  Rate Transition{1,3,6..7} (4 alike) : RateTransition  Integrity=off  Deterministic=off  OutPortSampleTime=0
  Setup1 : speedgoatlib/IO503/TEWS TPMC466 Internal blocks/Setup   port=1  transceiver=RS422  standard=on  baudrate=921600  bauddivisor=1  mode8x=16x (standard)  prescale=off  width=8  nstop=1  parity=None  rlevel=quarter full (16)  ctsmode=none  xonoff=none  xon=17  xoff=19  rs485mode=off  rs485delay=1  slot=brdslot
  Setup2 : speedgoatlib/IO503/TEWS TPMC466 Internal blocks/Setup   port=2  transceiver=RS485 half-duplex  standard=on  baudrate=2764800  bauddivisor=1  mode8x=16x (standard)  prescale=off  width=8  nstop=1  parity=None  rlevel=quarter full (16)  ctsmode=none  xonoff=XON/XOFF  xon=17  xoff=19  rs485mode=on  rs485delay=1  slot=brdslot
  Setup3 : speedgoatlib/IO503/TEWS TPMC466 Internal blocks/Setup   port=3  transceiver=RS485 half-duplex  standard=on  baudrate=115200  bauddivisor=1  mode8x=16x (standard)  prescale=off  width=8  nstop=1  parity=None  rlevel=half full (32)  ctsmode=none  xonoff=none  xon=17  xoff=19  rs485mode=off  rs485delay=0  slot=brdslot
  Setup4 : speedgoatlib/IO503/TEWS TPMC466 Internal blocks/Setup   port=4  transceiver=RS485 half-duplex  standard=on  baudrate=115200  bauddivisor=1  mode8x=16x (standard)  prescale=off  width=8  nstop=1  parity=None  rlevel=half full (32)  ctsmode=none  xonoff=none  xon=17  xoff=19  rs485mode=off  rs485delay=0  slot=brdslot
  Out1 : Outport
  Out2 : Outport  Port=2
  Out3 : Outport  Port=3
  Out4 : Outport  Port=4
  wires:
  RS232 ISR/4(Recv 4) -> Rate Transition7/1
  RS232 ISR/3(Recv 3) -> Rate Transition6/1
  Rate Transition7/1 -> Out4/1
  Rate Transition6/1 -> Out3/1
  Rate Transition5/1 -> RS232 ISR/4(Xmt 4)
  Rate Transition4/1 -> RS232 ISR/3(Xmt 3)
  FIFO write 4/1 -> Rate Transition5/1
  In4/1 -> FIFO write 4/1
  FIFO write 4/2 -> Enable TX 3/1
  FIFO write 3/1 -> Rate Transition4/1
  In3/1 -> FIFO write 3/1
  FIFO write 3/2 -> Enable TX 2/1
  Rate Transition1/1 -> Out1/1
  Rate Transition3/1 -> Out2/1
  Rate Transition/1 -> RS232 ISR/1(Xmt 1)
  Rate Transition2/1 -> RS232 ISR/2(Xmt 2)
  FIFO write 1/2 -> "Enable TX "/1
  IRQ Source/1 -> RS232 ISR/Trigger
  RS232 ISR/1(Recv 1) -> Rate Transition1/1
  RS232 ISR/2(Recv 2) -> Rate Transition3/1
  FIFO write 1/1 -> Rate Transition/1
  In1/1 -> FIFO write 1/1
  FIFO write 2/1 -> Rate Transition2/1
  In2/1 -> FIFO write 2/1
  FIFO write 2/2 -> Enable TX 1/1

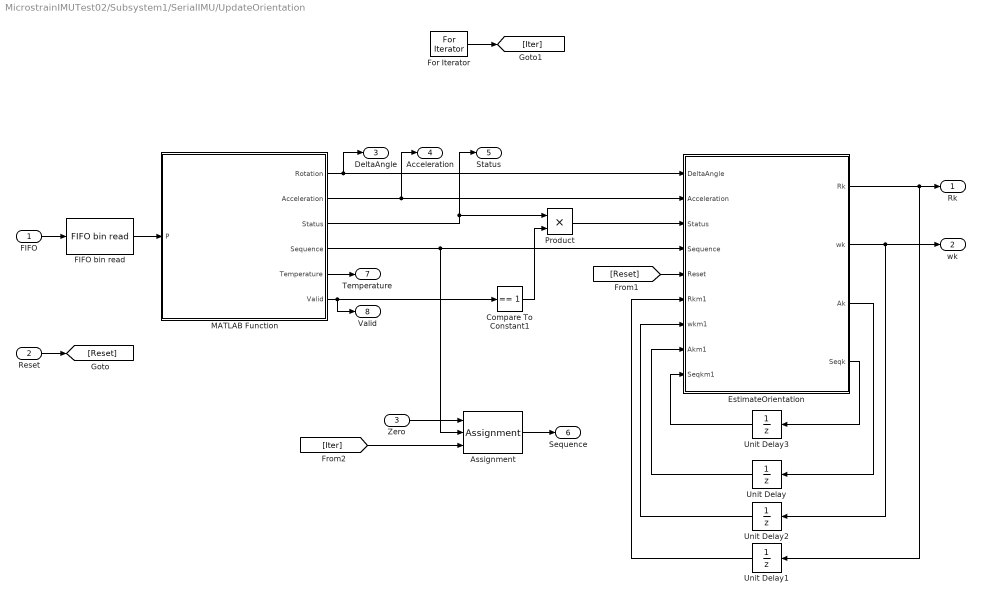
== system MicrostrainIMUTest02/Subsystem1/SerialIMU/UpdateOrientation ==
  FIFO : Inport
  Reset : Inport  Port=2
  Zero : Inport  Port=3
  Assignment : Assignment  IndexOptions=Index vector (port)  Indices=1  OutputSizes=1
  Compare To Constant1 : simulink/Logic and Bit Operations/Compare To Constant  relop===  const=1  OutDataTypeStr=uint8
  EstimateOrientation : MATLAB Function  TreatAsAtomicUnit=on
  "FIFO bin read " : xpcseriallib/FIFO bin read   header={char([254 129 255 85])}  lengths=[36]  hold=Zero output if no new data  enable=off  maxsize=36  outputtype=8 bit uint null terminated  sampletime=-1
  For Iterator : ForIterator
  MATLAB Function : MATLAB Function  TreatAsAtomicUnit=on
  Product : Product  RndMeth=Zero
  Unit Delay : UnitDelay  InitialCondition=[0; 0; 0]  SampleTime=-1
  Unit Delay1 : UnitDelay  InitialCondition=zeros(3,3)  SampleTime=-1
  Unit Delay2 : UnitDelay  InitialCondition=[0; 0; 0]  SampleTime=-1
  Unit Delay3 : UnitDelay  SampleTime=-1
  Rk : Outport  InitialOutput=zeros(3,3)
  wk : Outport  Port=2  InitialOutput=zeros(3,1)
  DeltaAngle : Outport  Port=3  InitialOutput=zeros(3,1)
  Acceleration : Outport  Port=4  InitialOutput=zeros(3,1)
  Status : Outport  Port=5  InitialOutput=0
  Sequence : Outport  Port=6  InitialOutput=[0; 0; 0; 0; 0]
  Temperature : Outport  Port=7  InitialOutput=0
  Valid : Outport  Port=8  InitialOutput=0
  wires:
  MATLAB Function/2(Acceleration) -> Acceleration/1, EstimateOrientation/2(Acceleration)
  MATLAB Function/1(Rotation) -> DeltaAngle/1, EstimateOrientation/1(DeltaAngle)
  MATLAB Function/3(Status) -> Status/1, Product/1
  MATLAB Function/4(Sequence) -> Assignment/2, EstimateOrientation/4(Sequence)
  MATLAB Function/5(Temperature) -> Temperature/1
  MATLAB Function/6(Valid) -> Valid/1, Compare To Constant1/1
  EstimateOrientation/3(Ak) -> Unit Delay/1
  Unit Delay/1 -> EstimateOrientation/8(Akm1)
  EstimateOrientation/1(Rk) -> Rk/1, Unit Delay1/1
  Unit Delay1/1 -> EstimateOrientation/6(Rkm1)
  [Reset] -> EstimateOrientation/5(Reset)
  Product/1 -> EstimateOrientation/3(Status)
  Compare To Constant1/1 -> Product/2
  FIFO/1 -> "FIFO bin read "/1
  EstimateOrientation/4(Seqk) -> Unit Delay3/1
  Unit Delay3/1 -> EstimateOrientation/9(Seqkm1)
  Reset/1 -> [Reset]
  "FIFO bin read "/1 -> MATLAB Function/1(P)
  [Iter] -> Assignment/3
  Assignment/1 -> Sequence/1
  Zero/1 -> Assignment/1
  For Iterator/1 -> [Iter]
  EstimateOrientation/2(wk) -> wk/1, Unit Delay2/1
  Unit Delay2/1 -> EstimateOrientation/7(wkm1)

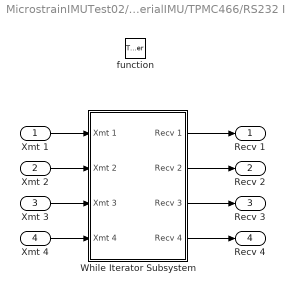
== system MicrostrainIMUTest02/Subsystem1/SerialIMU/TPMC466/RS232 ISR ==
  Xmt 1 : Inport
  Xmt 2 : Inport  Port=2
  Xmt 3 : Inport  Port=3
  Xmt 4 : Inport  Port=4
  function : TriggerPort  TriggerType=function-call
  While Iterator Subsystem : Subsystem  TreatAsAtomicUnit=on
  Recv 1 : Outport  SourceOfInitialOutputValue=Input signal
  Recv 2 : Outport  Port=2  SourceOfInitialOutputValue=Input signal
  Recv 3 : Outport  Port=3  SourceOfInitialOutputValue=Input signal
  Recv 4 : Outport  Port=4  SourceOfInitialOutputValue=Input signal
  wires:
  While Iterator Subsystem/4(Recv 4) -> Recv 4/1
  While Iterator Subsystem/3(Recv 3) -> Recv 3/1
  Xmt 4/1 -> While Iterator Subsystem/4(Xmt 4)
  Xmt 3/1 -> While Iterator Subsystem/3(Xmt 3)
  While Iterator Subsystem/2(Recv 2) -> Recv 2/1
  While Iterator Subsystem/1(Recv 1) -> Recv 1/1
  Xmt 2/1 -> While Iterator Subsystem/2(Xmt 2)
  Xmt 1/1 -> While Iterator Subsystem/1(Xmt 1)

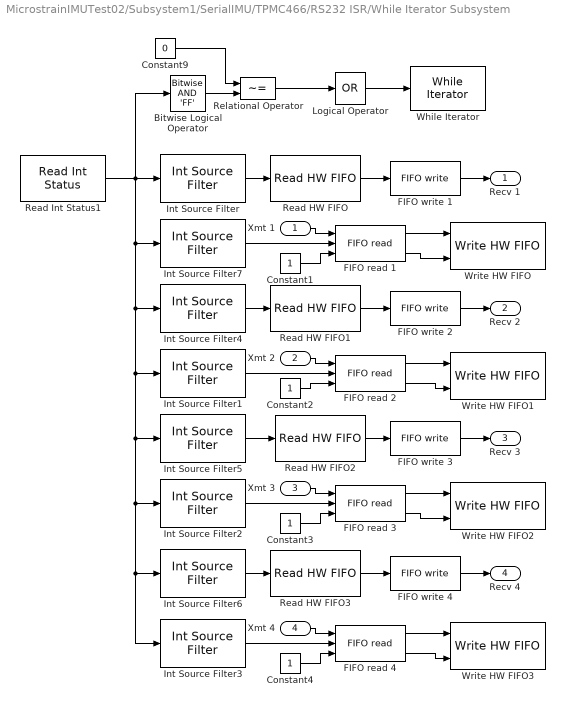
== system MicrostrainIMUTest02/Subsystem1/SerialIMU/TPMC466/RS232 ISR/While Iterator Subsystem ==
  Xmt 1 : Inport
  Xmt 2 : Inport  Port=2
  Xmt 3 : Inport  Port=3
  Xmt 4 : Inport  Port=4
  Bitwise Logical Operator : simulink/Logic and Bit Operations/Bitwise Operator  logicop=AND  UseBitMask=on  BitMask='FF'  BitMaskRealWorld=Stored Integer
  Constant{1..4} (4 alike) : Constant  OutDataTypeStr=uint32
  Constant9 : Constant  Value=0  OutDataTypeStr=uint32
  FIFO read {1..4} (4 alike) : xpcseriallib/FIFO read   maxsize=60  minsize=1  usedelimiter=off  delimiter=13  outputtype=count+32 bit uint  enable=on  enableout=on  sampletime=-1
  FIFO write 1 : xpcseriallib/FIFO write   size=1024  inputtype=count+32 bit uint  present=off  sampletime=-1  id=RCV channel 1, IRQ 9
  FIFO write 2 : xpcseriallib/FIFO write   size=1024  inputtype=count+32 bit uint  present=off  sampletime=-1  id=RCV channel 2, IRQ 9
  FIFO write 3 : xpcseriallib/FIFO write   size=1024  inputtype=count+32 bit uint  present=off  sampletime=-1  id=RCV channel 3, IRQ 9
  FIFO write 4 : xpcseriallib/FIFO write   size=1024  inputtype=count+32 bit uint  present=off  sampletime=-1  id=RCV channel 4, IRQ 9
  Int Source Filter : speedgoatlib/IO503/TEWS TPMC466 Internal blocks/Int Source Filter  port=1  value=Receive data
  Int Source Filter1 : speedgoatlib/IO503/TEWS TPMC466 Internal blocks/Int Source Filter  port=2  value=Transmitter empty
  Int Source Filter2 : speedgoatlib/IO503/TEWS TPMC466 Internal blocks/Int Source Filter  port=3  value=Transmitter empty
  Int Source Filter3 : speedgoatlib/IO503/TEWS TPMC466 Internal blocks/Int Source Filter  port=4  value=Transmitter empty
  Int Source Filter4 : speedgoatlib/IO503/TEWS TPMC466 Internal blocks/Int Source Filter  port=2  value=Receive data
  Int Source Filter5 : speedgoatlib/IO503/TEWS TPMC466 Internal blocks/Int Source Filter  port=3  value=Receive data
  Int Source Filter6 : speedgoatlib/IO503/TEWS TPMC466 Internal blocks/Int Source Filter  port=4  value=Receive data
  Int Source Filter7 : speedgoatlib/IO503/TEWS TPMC466 Internal blocks/Int Source Filter  port=1  value=Transmitter empty
  Logical Operator : Logic  Operator=OR  Inputs=1  AllPortsSameDT=off
  Read HW FIFO : speedgoatlib/IO503/TEWS TPMC466 Internal blocks/Read HW FIFO  port=1  flush=on  slot=subslot
  Read HW FIFO1 : speedgoatlib/IO503/TEWS TPMC466 Internal blocks/Read HW FIFO  port=2  flush=on  slot=subslot
  Read HW FIFO2 : speedgoatlib/IO503/TEWS TPMC466 Internal blocks/Read HW FIFO  port=3  flush=on  slot=subslot
  Read HW FIFO3 : speedgoatlib/IO503/TEWS TPMC466 Internal blocks/Read HW FIFO  port=4  flush=on  slot=subslot
  Read Int Status1 : speedgoatlib/IO503/TEWS TPMC466 Internal blocks/Read Int Status  slot=subslot
  Relational Operator : RelationalOperator  Operator=~=
  While Iterator : WhileIterator  MaxIters=65  WhileBlockType=do-while
  Write HW FIFO : speedgoatlib/IO503/TEWS TPMC466 Internal blocks/Write HW FIFO  port=1  slot=subslot
  Write HW FIFO1 : speedgoatlib/IO503/TEWS TPMC466 Internal blocks/Write HW FIFO  port=2  slot=subslot
  Write HW FIFO2 : speedgoatlib/IO503/TEWS TPMC466 Internal blocks/Write HW FIFO  port=3  slot=subslot
  Write HW FIFO3 : speedgoatlib/IO503/TEWS TPMC466 Internal blocks/Write HW FIFO  port=4  slot=subslot
  Recv 1 : Outport  SourceOfInitialOutputValue=Input signal
  Recv 2 : Outport  Port=2  SourceOfInitialOutputValue=Input signal
  Recv 3 : Outport  Port=3  SourceOfInitialOutputValue=Input signal
  Recv 4 : Outport  Port=4  SourceOfInitialOutputValue=Input signal
  wires:
  Read HW FIFO3/1 -> FIFO write 4/1
  FIFO write 4/1 -> Recv 4/1
  Read HW FIFO2/1 -> FIFO write 3/1
  FIFO write 3/1 -> Recv 3/1
  Int Source Filter6/1 -> Read HW FIFO3/1
  Int Source Filter5/1 -> Read HW FIFO2/1
  Constant3/1 -> FIFO read 3/3
  FIFO read 3/2 -> Write HW FIFO2/2
  FIFO read 3/1 -> Write HW FIFO2/1
  Xmt 3/1 -> FIFO read 3/1
  Int Source Filter2/1 -> FIFO read 3/2
  Constant2/1 -> FIFO read 2/3
  Constant1/1 -> FIFO read 1/3
  FIFO read 2/2 -> Write HW FIFO1/2
  FIFO read 1/2 -> Write HW FIFO/2
  FIFO read 1/1 -> Write HW FIFO/1
  FIFO read 2/1 -> Write HW FIFO1/1
  Xmt 2/1 -> FIFO read 2/1
  Int Source Filter1/1 -> FIFO read 2/2
  Read HW FIFO1/1 -> FIFO write 2/1
  FIFO write 2/1 -> Recv 2/1
  Int Source Filter4/1 -> Read HW FIFO1/1
  Xmt 1/1 -> FIFO read 1/1
  Int Source Filter7/1 -> FIFO read 1/2
  Read HW FIFO/1 -> FIFO write 1/1
  FIFO write 1/1 -> Recv 1/1
  Int Source Filter/1 -> Read HW FIFO/1
  Read Int Status1/1 -> Bitwise Logical Operator/1, Int Source Filter6/1, Int Source Filter3/1, Int Source Filter2/1, Int Source Filter5/1, Int Source Filter1/1, Int Source Filter4/1, Int Source Filter7/1, Int Source Filter/1
  Constant9/1 -> Relational Operator/1
  Bitwise Logical Operator/1 -> Relational Operator/2
  Relational Operator/1 -> Logical Operator/1
  Logical Operator/1 -> While Iterator/1
  Constant4/1 -> FIFO read 4/3
  FIFO read 4/2 -> Write HW FIFO3/2
  FIFO read 4/1 -> Write HW FIFO3/1
  Xmt 4/1 -> FIFO read 4/1
  Int Source Filter3/1 -> FIFO read 4/2

== matlab function MicrostrainIMUTest02/Subsystem1/UpdateOrientation/EstimateOrientation ==
  data: DeltaAngle input; Acceleration input; Status input; Sequence input; Reset input; Rk output; wk output; Rkm1 input; wkm1 input; Akm1 input; Ak output; Seqkm1 input; Seqk output
function [Rk, wk, Ak, Seqk] = fcn(DeltaAngle,Acceleration,Status,Sequence,Reset,Rkm1,wkm1,Akm1,Seqkm1) %#codegen
    [Rk, wk, Ak, Seqk] = estimateOrientation(DeltaAngle,Acceleration,Rkm1,wkm1,Akm1,Status,Sequence,Seqkm1,Reset);
end

== matlab function MicrostrainIMUTest02/Subsystem/MATLAB Function ==
  data: M input; Rk output; AngRate input; Accel input; wk output; ak output; timer output
function [Rk, wk, ak, timer] = fcn(M, AngRate, Accel)
    %#codegen
    Rk = double(reshape(typecast(M, 'single'), 3, 3).');
    wk = double(typecast(AngRate, 'single'));
    ak = double(typecast(Accel, 'single'));
    timer = double(M(1))/62500;
end

== matlab function MicrostrainIMUTest02/Subsystem1/ComputeEulerAngles ==
  data: RkIn input; wk input; RCal input; Reset input; R0In input; ZYX output; dZYX output; Rk output; R0 output; YawRolloverIn input; YawRollover output
function [ZYX, dZYX, Rk, R0, YawRollover] = fcn(RkIn, wk, RCal, Reset, R0In, YawRolloverIn) %#codegen
    % Convert from IMU frame to robot frame and compute Euler angles. The
    % yaw angle is zeroed whenever (Reset) is true.
        
    if (Reset)
        % Compute the rotation matrix which zeroes the initial yaw
        qT0 = M_to_ZYX(RkIn*RCal);
        R0  = Rz(-qT0(1));
    else
        R0 = R0In;
    end
    
    % Transform from IMU to robot frame and zero initial yaw
    Rk = R0*RkIn*RCal;
    
    % Convert Rk to ZYX Euler angles
    ZYX = M_to_ZYX(Rk);
    
    % Unroll yaw
    YawRolloverCount = YawRolloverIn(1);
    PreviousYaw      = YawRolloverIn(2);
    CurrentYaw       = ZYX(1);
    YawRolloverCount = YawRolloverCount + getYawRollover(CurrentYaw, PreviousYaw);
    YawRollover      = [YawRolloverCount; CurrentYaw];
    ZYX(1)           = ZYX(1) + 2*pi*YawRolloverCount;
    
    % Compute Euler angle derivatives
    qzT = ZYX(1);
    qyT = ZYX(2);
    
    if cos(qyT)>1e-3
        dZYX = [0 -sin(qzT) cos(qzT)*cos(qyT); 0 cos(qzT) sin(qzT)*cos(qyT); 1 0 -sin(qyT)]\(R0*RkIn*wk);
    else
        dZYX = [0; 0; 0];
    end
end

function R = Rz(t)
    R = [cos(t) -sin(t) 0; sin(t) cos(t) 0; 0 0 1];
end

function Rollover = getYawRollover(CurrentYaw, PreviousYaw)
    % Determine if a rollover has occurred on yaw angle If a rollover is
    % detected, the output Rollover is either +1 or -1, depending on the
    % direction of the rollover.
  
    if (PreviousYaw>0 && CurrentYaw < (PreviousYaw-pi))
        Rollover = 1;
    elseif (PreviousYaw<0 && CurrentYaw > (PreviousYaw+pi))
        Rollover = -1;
    else
        Rollover = 0;
    end
end
